simulink library "lib_energy_storage"  (Simulink 7.9)
settings: Solver=ode45  SolverMode=SingleTasking  StartTime=0.0  StopTime=10.0  RelTol=1e-3
undefined symbols (not defined in the file or in its folder): air_cp, amb_tmp, cyc_mph, enable_stop, ess_cap, ess_cap_scale, ess_cb, ess_cc, ess_coulombic_eff, ess_init_soc, ess_max_ah_cap, ess_max_p, ess_max_p_soc, ess_max_soc, ess_max_volts, ess_min_soc, ess_min_volts, ess_MMi, ess_MMo, ess_mod_airflow, ess_mod_cp, ess_mod_cpm, ess_mod_init_tmp, ess_module_mass, ess_module_num, ess_on, ess_parallel_mod_num, ess_r, ess_r_chg, ess_r_dis, ess_rc, ess_re, ess_res_scale_coef, ess_res_scale_fun, ess_rt, ess_set_tmp, ess_soc, ess_th_calc, ess_th_res, ess_th_res_off, ess_th_res_on, ess_tmp, ess_voc, fund_byu, fund_byuop, mc_min_volts, saber_air_temp, Saber_Battery_IO_File, saber_init_soc, saber_init_temp, saber_init_voc, saber_k_cb, saber_k_cc, saber_k_rc, saber_k_re, saber_k_rt, saber_k_soc, t_soc, time_step
libraries: lib_energy_storage x3
(part 2 of 3)

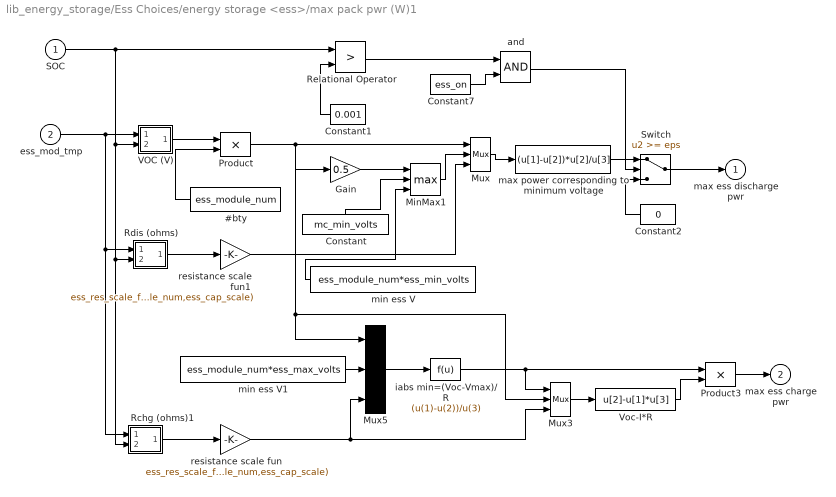
== system lib_energy_storage/Ess Choices/energy storage <ess>/max pack pwr (W)1 ==
  SOC : Inport
  ess_mod_tmp : Inport  Port=2
  #bty : Constant  Value=ess_module_num
  Constant : Constant  Value=mc_min_volts
  Constant1 : Constant  Value=0.001
  Constant2 : Constant  Value=0
  Constant7 : Constant  Value=ess_on
  Gain : Gain  Gain=0.5  SaturateOnIntegerOverflow=on  OutDataTypeStr=Inherit: Same as input  ParamDataTypeStr=Inherit: Same as input
  MinMax1 : MinMax  Function=max  Inputs=3  SaturateOnIntegerOverflow=on  InputSameDT=on
  Mux : Mux  Inputs=3
  Mux3 : Mux  Inputs=3
  Mux5 : Mux  Inputs=3
  Product : Product  SaturateOnIntegerOverflow=on  RndMeth=Zero  InputSameDT=on  OutDataTypeStr=Inherit: Same as first input
  Product3 : Product  SaturateOnIntegerOverflow=on  RndMeth=Zero  InputSameDT=on  OutDataTypeStr=Inherit: Same as first input
  Rchg (ohms)1 : Subsystem  mask(2-D Table Lookup){xindex=ess_tmp, yindex=ess_soc, table=ess_r_chg}
      mask prompts: xindex "X Index"; yindex "Y Index"
      mask help:
      | Two Dimensional Table Lookup
      | The first input corresponds to X Index and the second input corresponds to the Y Index
      mask init:
      | sftab2chk(xindex,yindex,table);
      mask Help: This block returns a linearly interpolated intersection from the table using the X index (which corresponds to the rows of the table) and the Y index (which corresponds to the columns of the table).  Extrapolation is used.
      mask Display: plot(-10,-10,110,110,[90,50,10],[90,40,30],[90,50,10],[50,26,20],[90,50,10],[22,13,10])
  Rdis (ohms) : Subsystem  mask(2-D Table Lookup){xindex=ess_tmp, yindex=ess_soc, table=ess_r_dis}
      mask prompts: xindex "X Index"; yindex "Y Index"
      mask help:
      | Two Dimensional Table Lookup
      | The first input corresponds to X Index and the second input corresponds to the Y Index
      mask init:
      | sftab2chk(xindex,yindex,table);
      mask Help: This block returns a linearly interpolated intersection from the table using the X index (which corresponds to the rows of the table) and the Y index (which corresponds to the columns of the table).  Extrapolation is used.
      mask Display: plot(-10,-10,110,110,[90,50,10],[90,40,30],[90,50,10],[50,26,20],[90,50,10],[22,13,10])
  Relational Operator : RelationalOperator  Operator=>  InputSameDT=on
  Switch : Switch  Threshold=eps  SaturateOnIntegerOverflow=on  InputSameDT=on
  VOC (V) : Subsystem  mask(2-D Table Lookup){xindex=ess_tmp, yindex=ess_soc, table=ess_voc}
      mask prompts: xindex "X Index"; yindex "Y Index"
      mask help:
      | Two Dimensional Table Lookup
      | The first input corresponds to X Index and the second input corresponds to the Y Index
      mask init:
      | sftab2chk(xindex,yindex,table);
      mask Help: This block returns a linearly interpolated intersection from the table using the X index (which corresponds to the rows of the table) and the Y index (which corresponds to the columns of the table).  Extrapolation is used.
      mask Display: plot(-10,-10,110,110,[90,50,10],[90,40,30],[90,50,10],[50,26,20],[90,50,10],[22,13,10])
  Voc-I*R : Fcn  Expr=u[2]-u[1]*u[3]
  and : Logic
  iabs min=(Voc-Vmax)/R : Fcn  Expr=(u(1)-u(2))/u(3)
  max power corresponding to minimum voltage : Fcn  Expr=(u[1]-u[2])*u[2]/u[3]
  min ess V : Constant  Value=ess_module_num*ess_min_volts
  min ess V1 : Constant  Value=ess_module_num*ess_max_volts
  resistance scale fun : Gain  Gain=ess_res_scale_fun(ess_res_scale_coef,ess_module_num,ess_cap_scale)  SaturateOnIntegerOverflow=on  OutDataTypeStr=Inherit: Same as input  ParamDataTypeStr=Inherit: Same as input
  resistance scale fun1 : Gain  Gain=ess_res_scale_fun(ess_res_scale_coef,ess_module_num,ess_cap_scale)  SaturateOnIntegerOverflow=on  OutDataTypeStr=Inherit: Same as input  ParamDataTypeStr=Inherit: Same as input
  max ess discharge pwr : Outport  InitialOutput=0
  max ess charge pwr : Outport  Port=2  InitialOutput=0
  wires:
  Constant7/1 -> and/2
  Relational Operator/1 -> and/1
  and/1 -> Switch/2
  min ess V/1 -> MinMax1/3
  ess_mod_tmp/1 -> VOC (V)/1(x0), Rdis (ohms)/1(x0), Rchg (ohms)1/1(x0)
  Constant1/1 -> Relational Operator/2
  Constant/1 -> MinMax1/2
  Mux/1 -> max power corresponding to minimum voltage/1
  Gain/1 -> MinMax1/1
  MinMax1/1 -> Mux/2
  Product/1 -> Mux/1, Gain/1, Mux5/1, Mux3/2
  resistance scale fun1/1 -> Mux/3
  VOC (V)/1(table out) -> Product/1
  Rdis (ohms)/1(table out) -> resistance scale fun1/1
  max power corresponding to minimum voltage/1 -> Switch/1
  Constant2/1 -> Switch/3
  SOC/1 -> Relational Operator/1, VOC (V)/2(y0), Rdis (ohms)/2(y0), Rchg (ohms)1/2(y0)
  Switch/1 -> max ess discharge pwr/1
  min ess V1/1 -> Mux5/2
  Mux5/1 -> iabs min=(Voc-Vmax)/R/1
  Mux3/1 -> Voc-I*R/1
  iabs min=(Voc-Vmax)/R/1 -> Mux3/1, Product3/1
  Voc-I*R/1 -> Product3/2
  Product3/1 -> max ess charge pwr/1
  resistance scale fun/1 -> Mux5/3, Mux3/3
  Rchg (ohms)1/1(table out) -> resistance scale fun/1
  #bty/1 -> Product/2

== system lib_energy_storage/Ess Choices/energy storage <ess>/pack Voc, Rint ==
  SOC (prev) : Inport
  req'd battery power (W) : Inport  Port=2
  mod tmp   (C) : Inport  Port=3
  #bty : Constant  Value=ess_module_num
  Product : Product  SaturateOnIntegerOverflow=on  RndMeth=Zero  InputSameDT=on  OutDataTypeStr=Inherit: Same as first input
  Rchg (ohms) : Subsystem  mask(2-D Table Lookup){xindex=ess_tmp, yindex=ess_soc, table=ess_r_chg}
      mask prompts: xindex "X Index"; yindex "Y Index"
      mask help:
      | Two Dimensional Table Lookup
      | The first input corresponds to X Index and the second input corresponds to the Y Index
      mask init:
      | sftab2chk(xindex,yindex,table);
      mask Help: This block returns a linearly interpolated intersection from the table using the X index (which corresponds to the rows of the table) and the Y index (which corresponds to the columns of the table).  Extrapolation is used.
      mask Display: plot(-10,-10,110,110,[90,50,10],[90,40,30],[90,50,10],[50,26,20],[90,50,10],[22,13,10])
  Rdis (ohms) : Subsystem  mask(2-D Table Lookup){xindex=ess_tmp, yindex=ess_soc, table=ess_r_dis}
      mask prompts: xindex "X Index"; yindex "Y Index"
      mask help:
      | Two Dimensional Table Lookup
      | The first input corresponds to X Index and the second input corresponds to the Y Index
      mask init:
      | sftab2chk(xindex,yindex,table);
      mask Help: This block returns a linearly interpolated intersection from the table using the X index (which corresponds to the rows of the table) and the Y index (which corresponds to the columns of the table).  Extrapolation is used.
      mask Display: plot(-10,-10,110,110,[90,50,10],[90,40,30],[90,50,10],[50,26,20],[90,50,10],[22,13,10])
  Switch : Switch  SaturateOnIntegerOverflow=on  InputSameDT=on
  VOC (V) : Subsystem  mask(2-D Table Lookup){xindex=ess_tmp, yindex=ess_soc, table=ess_voc}
      mask prompts: xindex "X Index"; yindex "Y Index"
      mask help:
      | Two Dimensional Table Lookup
      | The first input corresponds to X Index and the second input corresponds to the Y Index
      mask init:
      | sftab2chk(xindex,yindex,table);
      mask Help: This block returns a linearly interpolated intersection from the table using the X index (which corresponds to the rows of the table) and the Y index (which corresponds to the columns of the table).  Extrapolation is used.
      mask Display: plot(-10,-10,110,110,[90,50,10],[90,40,30],[90,50,10],[50,26,20],[90,50,10],[22,13,10])
  resistance scale fun : Gain  Gain=ess_res_scale_fun(ess_res_scale_coef,ess_module_num,ess_cap_scale)  SaturateOnIntegerOverflow=on  OutDataTypeStr=Inherit: Same as input  ParamDataTypeStr=Inherit: Same as input
  resistance scale fun1 : Gain  Gain=ess_res_scale_fun(ess_res_scale_coef,ess_module_num,ess_cap_scale)  SaturateOnIntegerOverflow=on  OutDataTypeStr=Inherit: Same as input  ParamDataTypeStr=Inherit: Same as input
  pack open- circuit voltage : Outport  InitialOutput=0
  pack resistance : Outport  Port=2  InitialOutput=0
  wires:
  mod tmp   (C)/1 -> Rchg (ohms)/1(x0), Rdis (ohms)/1(x0), VOC (V)/1(x0)
  SOC (prev)/1 -> Rchg (ohms)/2(y0), Rdis (ohms)/2(y0), VOC (V)/2(y0)
  req'd battery power (W)/1 -> Switch/2
  VOC (V)/1(table out) -> Product/1
  Product/1 -> pack open- circuit voltage/1
  #bty/1 -> Product/2
  Switch/1 -> pack resistance/1
  Rdis (ohms)/1(table out) -> resistance scale fun/1
  resistance scale fun/1 -> Switch/1
  Rchg (ohms)/1(table out) -> resistance scale fun1/1
  resistance scale fun1/1 -> Switch/3

== system lib_energy_storage/Ess Choices/energy storage <ess>/stop sim ==
  SOC : Inport
  Enable : EnablePort
  Const : Constant  Value=.001
  Relational Operator : RelationalOperator  Operator=<  InputSameDT=on
  Stop Simulation : Stop
  wires:
  Relational Operator/1 -> Stop Simulation/1
  SOC/1 -> Relational Operator/1
  Const/1 -> Relational Operator/2

== system lib_energy_storage/Ess Choices/energy storage <ess> RC/Allow simulation to stop based on  low SOC ==
  SOC : Inport
  Enable : EnablePort
  Const : Constant  Value=.001
  Relational Operator : RelationalOperator  Operator=<  InputSameDT=on
  Stop Simulation : Stop
  wires:
  Relational Operator/1 -> Stop Simulation/1
  SOC/1 -> Relational Operator/1
  Const/1 -> Relational Operator/2

== system lib_energy_storage/Ess Choices/energy storage <ess> RC/Block NOTES ==
  note: This block models the energy storage system as an SOC-dependent voltage
      | in series with an SOC- and current direction-dependent internal resistance.
      | SOC is computed assuming that A-h capacity is constant, but limited
      | such that a minimum voltage is never exceeded (replacing the
      | previous Peukert relationship which underpredicted battery capacity).
      |
      | Discharge power is limited here so as not to bring the bus (battery pack) voltage below
      | the minimum controller voltage or the minimum battery voltage and so as to allow
      | the solution of the quadratic eq'n for discharge current.
      |
      | Charge current is limited to ensure the voltage does not exceed a maximum
      | voltage
      |
      | Positive current is discharge current in the convention used here.
      | Power loss is computed as I*R+losses due to Coulombic (in)efficiency.
      |
      | Thermal modeling of the battery performance is modeled in the
      | OCV, Rint, and capacity.

== system lib_energy_storage/Ess Choices/energy storage <ess> RC/Model Parameters ==
  SOC : Inport
  Ess Temp : Inport  Port=2
  Preq : Inport  Port=3
  Terminator : Terminator
  cb : Lookup  InputValues=ess_tmp  Table=ess_cb  SaturateOnIntegerOverflow=on
  cc : Lookup  InputValues=ess_tmp  Table=ess_cc  SaturateOnIntegerOverflow=on
  rc : Subsystem  mask(2-D Table Lookup){xindex=ess_tmp, yindex=ess_soc, table=ess_rc}
      mask prompts: xindex "X Index"; yindex "Y Index"
      mask help:
      | Two Dimensional Table Lookup
      | The first input corresponds to X Index and the second input corresponds to the Y Index
      mask init:
      | sftab2chk(xindex,yindex,table);
      mask Help: This block returns a linearly interpolated intersection from the table using the X index (which corresponds to the rows of the table) and the Y index (which corresponds to the columns of the table).  Extrapolation is used.
      mask Display: plot(-10,-10,110,110,[90,50,10],[90,40,30],[90,50,10],[50,26,20],[90,50,10],[22,13,10])
  re : Subsystem  mask(2-D Table Lookup){xindex=ess_tmp, yindex=ess_soc, table=ess_re}
      mask prompts: xindex "X Index"; yindex "Y Index"
      mask help:
      | Two Dimensional Table Lookup
      | The first input corresponds to X Index and the second input corresponds to the Y Index
      mask init:
      | sftab2chk(xindex,yindex,table);
      mask Help: This block returns a linearly interpolated intersection from the table using the X index (which corresponds to the rows of the table) and the Y index (which corresponds to the columns of the table).  Extrapolation is used.
      mask Display: plot(-10,-10,110,110,[90,50,10],[90,40,30],[90,50,10],[50,26,20],[90,50,10],[22,13,10])
  rt : Subsystem  mask(2-D Table Lookup){xindex=ess_tmp, yindex=ess_soc, table=ess_rt}
      mask prompts: xindex "X Index"; yindex "Y Index"
      mask help:
      | Two Dimensional Table Lookup
      | The first input corresponds to X Index and the second input corresponds to the Y Index
      mask init:
      | sftab2chk(xindex,yindex,table);
      mask Help: This block returns a linearly interpolated intersection from the table using the X index (which corresponds to the rows of the table) and the Y index (which corresponds to the columns of the table).  Extrapolation is used.
      mask Display: plot(-10,-10,110,110,[90,50,10],[90,40,30],[90,50,10],[50,26,20],[90,50,10],[22,13,10])
  Cb : Outport  InitialOutput=0
  Cc : Outport  Port=2  InitialOutput=0
  Re : Outport  Port=3  InitialOutput=0
  Rc : Outport  Port=4  InitialOutput=0
  Rt : Outport  Port=5  InitialOutput=0
  wires:
  rc/1(table out) -> Rc/1
  rt/1(table out) -> Rt/1
  re/1(table out) -> Re/1
  cc/1 -> Cc/1
  cb/1 -> Cb/1
  SOC/1 -> rt/2(y0), rc/2(y0), re/2(y0)
  Preq/1 -> Terminator/1
  Ess Temp/1 -> rt/1(x0), rc/1(x0), re/1(x0), cc/1, cb/1

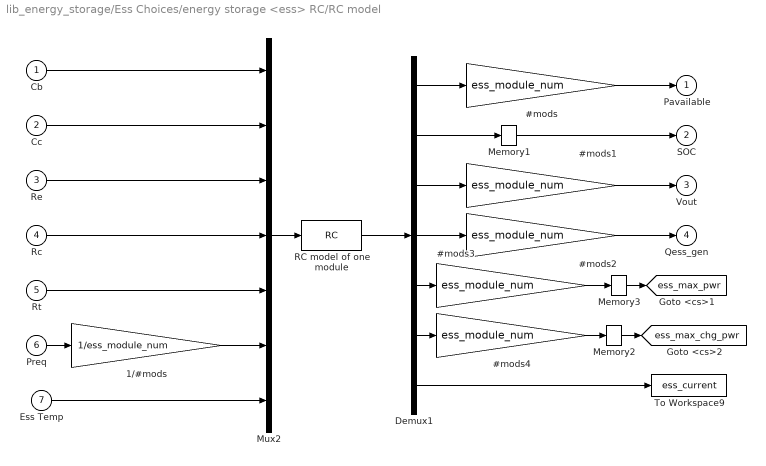
== system lib_energy_storage/Ess Choices/energy storage <ess> RC/RC model ==
  Cb : Inport
  Cc : Inport  Port=2
  Re : Inport  Port=3
  Rc : Inport  Port=4
  Rt : Inport  Port=5
  Preq : Inport  Port=6
  Ess Temp : Inport  Port=7
  #mods{,1..4} (5 alike) : Gain  Gain=ess_module_num  SaturateOnIntegerOverflow=on  OutDataTypeStr=Inherit: Same as input  ParamDataTypeStr=Inherit: Same as input
  1/#mods : Gain  Gain=1/ess_module_num  SaturateOnIntegerOverflow=on  OutDataTypeStr=Inherit: Same as input  ParamDataTypeStr=Inherit: Same as input
  Demux1 : Demux  Outputs=7
  Memory1 : Memory  X0=ess_init_soc
  Memory2 : Memory
  Memory3 : Memory
  Mux2 : Mux  Inputs=7
  RC model of one module : S-Function  FunctionName=RC  Parameters=ess_min_volts,ess_max_volts,mc_min_volts/ess_module_num,ess_soc,ess_tmp,ess_voc,ess_init_soc,ess_mod_init_tmp  EnableBusSupport=off
  To Workspace9 : ToWorkspace  VariableName=ess_current  SampleTime=-1
  Pavailable : Outport  InitialOutput=0
  SOC : Outport  Port=2  InitialOutput=0
  Vout : Outport  Port=3  InitialOutput=0
  Qess_gen : Outport  Port=4  InitialOutput=0
  tag scope: ess_max_chg_pwr=global, ess_max_pwr=global
  wires:
  RC model of one module/1 -> Demux1/1
  #mods2/1 -> Qess_gen/1
  Demux1/4 -> #mods2/1
  #mods1/1 -> Vout/1
  Demux1/3 -> #mods1/1
  #mods/1 -> Pavailable/1
  Demux1/1 -> #mods/1
  1/#mods/1 -> Mux2/6
  Preq/1 -> 1/#mods/1
  Mux2/1 -> RC model of one module/1
  Rt/1 -> Mux2/5
  Rc/1 -> Mux2/4
  Re/1 -> Mux2/3
  Cc/1 -> Mux2/2
  Cb/1 -> Mux2/1
  Ess Temp/1 -> Mux2/7
  Demux1/7 -> To Workspace9/1
  Demux1/6 -> #mods4/1
  Memory2/1 -> [ess_max_chg_pwr]
  Demux1/5 -> #mods3/1
  Memory3/1 -> [ess_max_pwr]
  Demux1/2 -> Memory1/1
  Memory1/1 -> SOC/1
  #mods3/1 -> Memory3/1
  #mods4/1 -> Memory2/1

== system lib_energy_storage/Ess Choices/energy storage <ess> RC/Thermal Model of Battery ==
  Qess_gen : Inport
  Enable : EnablePort  StatesWhenEnabling=reset
  #of mods : Gain  Gain=ess_module_num  SaturateOnIntegerOverflow=on  OutDataTypeStr=Inherit: Same as input  ParamDataTypeStr=Inherit: Same as input
  1/#of mods : Gain  Gain=1/ess_module_num  SaturateOnIntegerOverflow=on  OutDataTypeStr=Inherit: Same as input  ParamDataTypeStr=Inherit: Same as input
  1/mcp : Gain  Gain=1/(ess_module_mass*ess_mod_cp)  SaturateOnIntegerOverflow=on  OutDataTypeStr=Inherit: Same as input  ParamDataTypeStr=Inherit: Same as input
  Block NOTES : Subsystem
      mask Display: disp('Block\nNOTES')
  Memory : Memory  X0=cyc_mph(1,2)*.447
  Memory1 : Memory  X0=cyc_mph(1,2)*.447
  Mux20 : Mux  Inputs=3
  Qc : Sum  SaturateOnIntegerOverflow=on  InputSameDT=on  OutDataTypeStr=Inherit: Same as first input
  Qess_case : Fcn  Expr=(u(2) - u(1))/u(3)
  Saturation3 : Saturate  UpperLimit=1  LowerLimit=0
  Tair,ave : Subsystem  TreatAsAtomicUnit=on
  Tess2 : Integrator  InitialCondition=ess_mod_init_tmp
  thermostat : Fcn  Expr=u(1) - ess_set_tmp
  Tess : Outport  InitialOutput=0
  Tair : Outport  Port=2
  Qair : Outport  Port=3  OutputWhenDisabled=reset  InitialOutput=0
  wires:
  Tair,ave/1(Tair_ave) -> Tair/1, Mux20/2
  Tair,ave/2(Th Res) -> Mux20/3
  Mux20/1 -> Qess_case/1
  #of mods/1 -> Qair/1
  Memory/1 -> Tair,ave/1(Qess_case)
  Memory1/1 -> Tair,ave/Enable
  Saturation3/1 -> Memory1/1
  thermostat/1 -> Saturation3/1
  1/#of mods/1 -> Qc/2
  Qess_gen/1 -> 1/#of mods/1
  Tess2/1 -> thermostat/1, Mux20/1, Tess/1
  1/mcp/1 -> Tess2/1
  Qess_case/1 -> #of mods/1, Memory/1, Qc/1
  Qc/1 -> 1/mcp/1

== system lib_energy_storage/Ess Choices/energy storage <ess> RC/documentation9 ==

== system lib_energy_storage/Ess Choices/energy storage <ess> nnet/Limits ==
  power req : Inport
  power  available from battery : Inport  Port=2
  Const{1..4} (4 alike) : Constant  Value=0
  Relational Operator1 : RelationalOperator  Operator===  InputSameDT=on
  limited by battery : Logic  Operator=NOT  Inputs=1
  tag scope: ess_maxV_limited=global, ess_minV_limited=global, ess_pwr_limited=global, ess_soc_limited=global, mc_voltage_limited=global
  wires:
  Relational Operator1/1 -> limited by battery/1
  limited by battery/1 -> [ess_pwr_limited]
  power req/1 -> Relational Operator1/1
  power  available from battery/1 -> Relational Operator1/2
  Const4/1 -> [mc_voltage_limited]
  Const3/1 -> [ess_minV_limited]
  Const2/1 -> [ess_maxV_limited]
  Const1/1 -> [ess_soc_limited]

== system lib_energy_storage/Ess Choices/energy storage <ess> nnet/NNet ==
  Preq : Inport
  SOC : Inport  Port=2
  Enable : EnablePort
  De-Normalizer1 Voltage : Fcn  Expr=(u-0.2)*(ess_MMo(2,2)-ess_MMo(2,1))/(0.8-0.2)+ess_MMo(2,1)
  De-Normalizer2 Current : Fcn  Expr=(u-0.2)*(ess_MMo(1,2)-ess_MMo(1,1))/(0.8-0.2)+ess_MMo(1,1)
  Demux : Demux  Outputs=2
  Mux : Mux  Inputs=2
  Neural Network : Subsystem
  Normalizer Power : Fcn  Expr=(u-ess_MMi(1,1))/(ess_MMi(1,2)-ess_MMi(1,1))
  Normalizer SOC : Fcn  Expr=(u-ess_MMi(2,1))/(ess_MMi(2,2)-ess_MMi(2,1))
  V : Outport  InitialOutput=0
  i : Outport  Port=2  OutputWhenDisabled=reset  InitialOutput=0
  wires:
  De-Normalizer1 Voltage/1 -> V/1
  Demux/2 -> De-Normalizer1 Voltage/1
  Demux/1 -> De-Normalizer2 Current/1
  De-Normalizer2 Current/1 -> i/1
  Normalizer SOC/1 -> Mux/2
  SOC/1 -> Normalizer SOC/1
  Normalizer Power/1 -> Mux/1
  Preq/1 -> Normalizer Power/1
  Neural Network/1("y{1}") -> Demux/1
  Mux/1 -> Neural Network/1("p{1}")

== system lib_energy_storage/Ess Choices/energy storage <ess> nnet/No Thermal model ==
  Const1 : Constant  Value=0
  Const2 : Constant  Value=amb_tmp
  Const3 : Constant  Value=0
  To WS1 : ToWorkspace  VariableName=ess_pwr_loss_a
  To WS2 : ToWorkspace  VariableName=ess_mod_tmp
  To WS3 : ToWorkspace  VariableName=ess_air_tmp
  To WS4 : ToWorkspace  VariableName=ess_air_th_pwr
  wires:
  Const3/1 -> To WS4/1
  Const2/1 -> To WS3/1, To WS2/1
  Const1/1 -> To WS1/1

== system lib_energy_storage/Ess Choices/energy storage <ess> nnet/SOC algorithm ==
  note: SOC=(Max Ah capacity-Ah used)/Max Ah capacity
  (A) : Inport
  tmp (C) : Inport  Port=2
  (sec->hrs) : Gain  Gain=1/3600  SaturateOnIntegerOverflow=on  OutDataTypeStr=Inherit: Same as input  ParamDataTypeStr=Inherit: Same as input
  0 <= SOC <= 1 : Saturate  UpperLimit=1  LowerLimit=0
  A-h remaining : Sum  Inputs=-+  SaturateOnIntegerOverflow=on  InputSameDT=on  OutDataTypeStr=Inherit: Same as first input
  Ah used : Integrator  InitialConditionSource=external  InitialCondition=(1-ess_init_soc)*ess_max_ah_cap
  Fcn : Fcn  Expr=1/u
  Fcn1 : Fcn  Expr=(1-ess_init_soc)*u
  SOC : Product  SaturateOnIntegerOverflow=on  RndMeth=Zero  InputSameDT=on  OutDataTypeStr=Inherit: Same as first input
  Switch : Switch  SaturateOnIntegerOverflow=on  InputSameDT=on
  adjusted A : Product  SaturateOnIntegerOverflow=on  RndMeth=Zero  InputSameDT=on  OutDataTypeStr=Inherit: Same as first input
  coul eff : Lookup  InputValues=ess_tmp  Table=ess_coulombic_eff  SaturateOnIntegerOverflow=on
  max cap : Lookup  InputValues=ess_tmp  Table=ess_max_ah_cap  SaturateOnIntegerOverflow=on
  SOC1 : Outport  InitialOutput=0
  wires:
  Fcn1/1 -> Ah used/2
  max cap/1 -> Fcn1/1, Fcn/1, A-h remaining/2
  adjusted A/1 -> Switch/3
  coul eff/1 -> adjusted A/2
  tmp (C)/1 -> coul eff/1, max cap/1
  0 <= SOC <= 1/1 -> SOC1/1
  A-h remaining/1 -> SOC/1
  SOC/1 -> 0 <= SOC <= 1/1
  Fcn/1 -> SOC/2
  Ah used/1 -> A-h remaining/1
  (sec->hrs)/1 -> Ah used/1
  Switch/1 -> (sec->hrs)/1
  (A)/1 -> adjusted A/1, Switch/1, Switch/2

== system lib_energy_storage/Ess Choices/energy storage <ess> nnet/max pack pwr (W) ==
  SOC : Inport
  # batteries : Gain  Gain=ess_module_num  SaturateOnIntegerOverflow=on  OutDataTypeStr=Inherit: Same as input  ParamDataTypeStr=Inherit: Same as input
  max power : Lookup  InputValues=ess_max_p_soc  Table=ess_max_p  SaturateOnIntegerOverflow=on
  ess discharge pwr : Outport  InitialOutput=0
  wires:
  # batteries/1 -> ess discharge pwr/1
  max power/1 -> # batteries/1
  SOC/1 -> max power/1

== system lib_energy_storage/Ess Choices/energy storage <ess> nnet/stop sim ==
  SOC : Inport
  Enable : EnablePort
  Const : Constant  Value=.001
  Relational Operator : RelationalOperator  Operator=<  InputSameDT=on
  Stop Simulation : Stop
  wires:
  Relational Operator/1 -> Stop Simulation/1
  SOC/1 -> Relational Operator/1
  Const/1 -> Relational Operator/2

== system lib_energy_storage/Ess Choices/energy storage <ess> Saber/Block NOTES ==
  note: Saber co-simulation

== system lib_energy_storage/Ess Choices/energy storage <ess> Saber/Power ==
  Current : Inport
  Voltage : Inport  Port=2
  P=i*V : Product  SaturateOnIntegerOverflow=on  RndMeth=Zero  InputSameDT=on  OutDataTypeStr=Inherit: Same as first input
  To Workspace9 : ToWorkspace  VariableName=ess_pwr_out_a  SampleTime=-1
  Avail Power : Outport
  wires:
  P=i*V/1 -> Avail Power/1, To Workspace9/1
  Current/1 -> P=i*V/1
  Voltage/1 -> P=i*V/2

== system lib_energy_storage/Ess Choices/energy storage <ess> Saber/Power request ==
  power req'd : Inport
  1/# batteries : Gain  Gain=1/ess_module_num  SaturateOnIntegerOverflow=on  OutDataTypeStr=Inherit: Same as input  ParamDataTypeStr=Inherit: Same as input
  Relational Operator1 : RelationalOperator  Operator===  InputSameDT=on
  To Workspace8 : ToWorkspace  VariableName=ess_pwr_out_r  SampleTime=-1
  if P==0 : Constant  Value=0
  "if P==0, pass  P=0.0001" : Switch  Threshold=0.1  SaturateOnIntegerOverflow=on  InputSameDT=on
  non-zero power : Constant  Value=0.0001
  P request : Outport
  wires:
  power req'd/1 -> To Workspace8/1, 1/# batteries/1
  1/# batteries/1 -> "if P==0, pass  P=0.0001"/3, Relational Operator1/2
  "if P==0, pass  P=0.0001"/1 -> P request/1
  if P==0/1 -> Relational Operator1/1
  non-zero power/1 -> "if P==0, pass  P=0.0001"/1
  Relational Operator1/1 -> "if P==0, pass  P=0.0001"/2

== system lib_energy_storage/Ess Choices/energy storage <ess> Saber/SOC's ==
  Saber SOC's : Inport
  Const : Constant  Value=enable_stop
  Mean : Subsystem
  To Workspace2 : ToWorkspace  VariableName=saber_ess_SOC  SampleTime=-1
  soc mem : Memory  X0=ess_init_soc
  stop sim : Subsystem  TreatAsAtomicUnit=on
  tag scope: SOC=global
  wires:
  Saber SOC's/1 -> Mean/1(In), To Workspace2/1
  Const/1 -> stop sim/Enable
  Mean/1(Out) -> soc mem/1
  soc mem/1 -> [SOC], stop sim/1(SOC)

== system lib_energy_storage/Ess Choices/energy storage <ess> Saber/Temps ==
  Saber Temps : Inport
  Mean : Subsystem
  To WS2 : ToWorkspace  VariableName=ess_mod_tmp
  To Workspace3 : ToWorkspace  VariableName=saber_ess_temp  SampleTime=-1
  wires:
  Saber Temps/1 -> Mean/1(In), To Workspace3/1
  Mean/1(Out) -> To WS2/1

== system lib_energy_storage/Ess Choices/energy storage <ess> Saber/Thermal Power ==
  Saber Thermal P : Inport
  # batteries : Gain  Gain=ess_module_num  SaturateOnIntegerOverflow=on  OutDataTypeStr=Inherit: Same as input  ParamDataTypeStr=Inherit: Same as input
  Saturation : Saturate  UpperLimit=inf  LowerLimit=0
  Sum2 : Sum  Inputs=1  SaturateOnIntegerOverflow=on  InputSameDT=on  OutDataTypeStr=Inherit: Same as first input
  To Workspace3 : ToWorkspace  VariableName=saber_ess_th_pwr  SampleTime=-1
  To Workspace9 : ToWorkspace  VariableName=ess_pwr_loss_a  SampleTime=-1
  wires:
  Sum2/1 -> To Workspace9/1
  # batteries/1 -> Sum2/1, To Workspace3/1
  Saber Thermal P/1 -> Saturation/1
  Saturation/1 -> # batteries/1

== system lib_energy_storage/Ess Choices/energy storage <ess> Saber/Time Dependent Power Request ==
  P request : Inport
  Constant : Constant  Value=0
  Enabled Subsystem1 : Subsystem  TreatAsAtomicUnit=on
  IC : InitialCondition  Value=time_step
  Matrix Concatenation1 : lib_energy_storage/Ess Choices/energy storage <ess> Saber/Matrix Concatenation1  numInports=6  catMethod=Horizontal
  Memory1 : Memory  X0=.001  InheritSampleTime=on
  Memory2 : Memory  X0=80  InheritSampleTime=on
  Relational Operator : RelationalOperator  Operator===  InputSameDT=on
  Saturation : Saturate  UpperLimit=inf  LowerLimit=.001
  P request time : Outport
  wires:
  Relational Operator/1 -> Enabled Subsystem1/Enable
  [time] -> Relational Operator/2
  Enabled Subsystem1/1(Out1) -> Matrix Concatenation1/2
  Memory2/1 -> Matrix Concatenation1/4
  Matrix Concatenation1/1 -> P request time/1
  IC/1 -> Matrix Concatenation1/5
  Saturation/1 -> Memory1/1
  [time] -> Saturation/1
  Memory1/1 -> Matrix Concatenation1/3
  [time] -> IC/1
  Constant/1 -> Relational Operator/1, Matrix Concatenation1/1
  P request/1 -> Memory2/1, Matrix Concatenation1/6, Enabled Subsystem1/1(In1)  "P request"

== system lib_energy_storage/Ess Choices/energy storage <ess> Saber/Voltages ==
  Saber Voltages : Inport
  # batteries : Gain  Gain=ess_module_num  SaturateOnIntegerOverflow=on  OutDataTypeStr=Inherit: Same as input  ParamDataTypeStr=Inherit: Same as input
  Sum : Sum  Inputs=1  SaturateOnIntegerOverflow=on  InputSameDT=on  OutDataTypeStr=Inherit: Same as first input
  To Workspace1 : ToWorkspace  VariableName=ess_voltage  SampleTime=-1
  To Workspace11 : ToWorkspace  VariableName=saber_ess_voltage  SampleTime=-1
  ADV Voltage : Outport
  tag scope: bus_voltage=global
  wires:
  # batteries/1 -> Sum/1, To Workspace11/1
  Sum/1 -> [bus_voltage], To Workspace1/1, ADV Voltage/1
  Saber Voltages/1 -> # batteries/1

== system lib_energy_storage/Ess Choices/energy storage <ess> Saber/max pack pwr (W) ==
  note: Edit in the future
      | Used in series power follower
  Ground : Ground
  tag scope: ess_max_pwr=global
  wires:
  Ground/1 -> [ess_max_pwr]

== system lib_energy_storage/Ess Choices/energy storage <ess> fundamental model/Block NOTES ==
  note: Fundamentally based SOC model developed at BYU
      | Files needed:
      | input1.dat
      | input2.dat
      | input3.dat
      | nrel13cs.dll

== system lib_energy_storage/Ess Choices/energy storage <ess> fundamental model/ess tmp ==
  Qess_gen : Inport
  Enable : EnablePort  StatesWhenEnabling=reset
  #of mods : Gain  Gain=ess_module_num  SaturateOnIntegerOverflow=on  OutDataTypeStr=Inherit: Same as input  ParamDataTypeStr=Inherit: Same as input
  1/#of mods : Gain  Gain=1/ess_module_num  SaturateOnIntegerOverflow=on  OutDataTypeStr=Inherit: Same as input  ParamDataTypeStr=Inherit: Same as input
  1/mcp : Gain  Gain=1/(ess_module_mass*ess_mod_cp)  SaturateOnIntegerOverflow=on  OutDataTypeStr=Inherit: Same as input  ParamDataTypeStr=Inherit: Same as input
  Block NOTES : Subsystem
      mask Display: disp('Block\nNOTES')
  Memory : Memory  X0=cyc_mph(1,2)*.447
  Memory1 : Memory  X0=cyc_mph(1,2)*.447
  Mux20 : Mux  Inputs=3
  Qc : Sum  SaturateOnIntegerOverflow=on  InputSameDT=on  OutDataTypeStr=Inherit: Same as first input
  Qess_case : Fcn  Expr=(u(2) - u(1))/u(3)
  Saturation3 : Saturate  UpperLimit=1  LowerLimit=0
  Tair,ave : Subsystem  TreatAsAtomicUnit=on
  Tess2 : Integrator  InitialCondition=ess_mod_init_tmp
  thermostat : Fcn  Expr=u(1) - ess_set_tmp
  Tess : Outport  InitialOutput=0
  Tair : Outport  Port=2
  Qair : Outport  Port=3  OutputWhenDisabled=reset  InitialOutput=0
  wires:
  Tair,ave/1(Tair_ave) -> Tair/1, Mux20/2
  Tair,ave/2(Th Res) -> Mux20/3
  Mux20/1 -> Qess_case/1
  #of mods/1 -> Qair/1
  Memory/1 -> Tair,ave/1(Qess_case)
  Memory1/1 -> Tair,ave/Enable
  Saturation3/1 -> Memory1/1
  thermostat/1 -> Saturation3/1
  1/#of mods/1 -> Qc/2
  Qess_gen/1 -> 1/#of mods/1
  Tess2/1 -> thermostat/1, Mux20/1, Tess/1
  1/mcp/1 -> Tess2/1
  Qess_case/1 -> #of mods/1, Memory/1, Qc/1
  Qc/1 -> 1/mcp/1

== system lib_energy_storage/Ess Choices/energy storage <ess> fundamental model/max pack pwr (W) ==
  SOC : Inport
  # batteries : Gain  Gain=ess_module_num  SaturateOnIntegerOverflow=on  OutDataTypeStr=Inherit: Same as input  ParamDataTypeStr=Inherit: Same as input
  max power : Lookup  InputValues=ess_max_p_soc  Table=ess_max_p  SaturateOnIntegerOverflow=on
  ess discharge pwr : Outport  InitialOutput=0
  wires:
  # batteries/1 -> ess discharge pwr/1
  max power/1 -> # batteries/1
  SOC/1 -> max power/1

== system lib_energy_storage/Ess Choices/energy storage <ess> fundamental model/stop sim ==
  SOC : Inport
  Enable : EnablePort
  Const : Constant  Value=0.1
  Relational Operator : RelationalOperator  Operator=<  InputSameDT=on
  Stop Simulation : Stop
  wires:
  Relational Operator/1 -> Stop Simulation/1
  SOC/1 -> Relational Operator/1
  Const/1 -> Relational Operator/2

== system lib_energy_storage/Ess Choices/energy storage <ess> optima fundamental model/Block NOTES ==
  note: Fundamentally based SOC model developed at BYU
      | Files needed:
      | input1.dat
      | input2.dat
      | input3.dat
      | nrel13cs.dll

== system lib_energy_storage/Ess Choices/energy storage <ess> optima fundamental model/ess tmp ==
  Qess_gen : Inport
  Enable : EnablePort  StatesWhenEnabling=reset
  #of mods : Gain  Gain=ess_module_num  SaturateOnIntegerOverflow=on  OutDataTypeStr=Inherit: Same as input  ParamDataTypeStr=Inherit: Same as input
  1/#of mods : Gain  Gain=1/ess_module_num  SaturateOnIntegerOverflow=on  OutDataTypeStr=Inherit: Same as input  ParamDataTypeStr=Inherit: Same as input
  1/mcp : Gain  Gain=1/(ess_module_mass*ess_mod_cp)  SaturateOnIntegerOverflow=on  OutDataTypeStr=Inherit: Same as input  ParamDataTypeStr=Inherit: Same as input
  Block NOTES : Subsystem
      mask Display: disp('Block\nNOTES')
  Memory : Memory  X0=cyc_mph(1,2)*.447
  Memory1 : Memory  X0=cyc_mph(1,2)*.447
  Mux20 : Mux  Inputs=3
  Qc : Sum  SaturateOnIntegerOverflow=on  InputSameDT=on  OutDataTypeStr=Inherit: Same as first input
  Qess_case : Fcn  Expr=(u(2) - u(1))/u(3)
  Saturation3 : Saturate  UpperLimit=1  LowerLimit=0
  Tair,ave : Subsystem  TreatAsAtomicUnit=on
  Tess2 : Integrator  InitialCondition=ess_mod_init_tmp
  thermostat : Fcn  Expr=u(1) - ess_set_tmp
  Tess : Outport  InitialOutput=0
  Tair : Outport  Port=2
  Qair : Outport  Port=3  OutputWhenDisabled=reset  InitialOutput=0
  wires:
  Tair,ave/1(Tair_ave) -> Tair/1, Mux20/2
  Tair,ave/2(Th Res) -> Mux20/3
  Mux20/1 -> Qess_case/1
  #of mods/1 -> Qair/1
  Memory/1 -> Tair,ave/1(Qess_case)
  Memory1/1 -> Tair,ave/Enable
  Saturation3/1 -> Memory1/1
  thermostat/1 -> Saturation3/1
  1/#of mods/1 -> Qc/2
  Qess_gen/1 -> 1/#of mods/1
  Tess2/1 -> thermostat/1, Mux20/1, Tess/1
  1/mcp/1 -> Tess2/1
  Qess_case/1 -> #of mods/1, Memory/1, Qc/1
  Qc/1 -> 1/mcp/1

== system lib_energy_storage/Ess Choices/energy storage <ess> optima fundamental model/max pack pwr (W) ==
  SOC : Inport
  # batteries : Gain  Gain=ess_module_num  SaturateOnIntegerOverflow=on  OutDataTypeStr=Inherit: Same as input  ParamDataTypeStr=Inherit: Same as input
  max power : Lookup  InputValues=ess_max_p_soc  Table=ess_max_p  SaturateOnIntegerOverflow=on
  ess discharge pwr : Outport  InitialOutput=0
  wires:
  # batteries/1 -> ess discharge pwr/1
  max power/1 -> # batteries/1
  SOC/1 -> max power/1

== system lib_energy_storage/Ess Choices/energy storage <ess> optima fundamental model/stop sim ==
  SOC : Inport
  Enable : EnablePort
  Const : Constant  Value=.001
  Relational Operator : RelationalOperator  Operator=<  InputSameDT=on
  Stop Simulation : Stop
  wires:
  Relational Operator/1 -> Stop Simulation/1
  SOC/1 -> Relational Operator/1
  Const/1 -> Relational Operator/2

== system lib_energy_storage/Ess Choices/Ultracapacitor  System/Calc Iout/SOC limit ==
  SOC : Inport
  Pbty : Inport  Port=2
  Constant1 : Constant  Value=0.001
  Constant5 : Constant  Value=.999
  Constant9 : Constant  Value=0
  Logical Operator : Logic  Operator=OR
  Logical Operator1 : Logic
  Logical Operator2 : Logic  Operator=NOT  Inputs=1
  Relational Operator : RelationalOperator  Operator=>  InputSameDT=on
  Relational Operator3 : RelationalOperator  Operator=<  InputSameDT=on
  SOC>=.999 : RelationalOperator  InputSameDT=on
  charging (Preq is neg) : RelationalOperator  Operator=<  InputSameDT=on
  no power req if SOC<0 and trying  to discharge : Switch  Threshold=eps  SaturateOnIntegerOverflow=on  InputSameDT=on
  no power req if SOC>.999 and trying  to charge : Switch  Threshold=eps  SaturateOnIntegerOverflow=on  InputSameDT=on
  "Pbty, limited" : Outport  InitialOutput=0
  tag scope: ess_soc_hi_limited=global, ess_soc_low_limited=global
  wires:
  Constant1/1 -> Relational Operator/2
  Pbty/1 -> Relational Operator3/1, charging (Preq is neg)/1, no power req if SOC<0 and trying  to discharge/1
  Logical Operator/1 -> Logical Operator2/1, no power req if SOC<0 and trying  to discharge/2
  SOC/1 -> Relational Operator/1, SOC>=.999/1
  SOC>=.999/1 -> Logical Operator1/1
  charging (Preq is neg)/1 -> Logical Operator1/2
  Constant5/1 -> SOC>=.999/2
  no power req if SOC<0 and trying  to discharge/1 -> no power req if SOC>.999 and trying  to charge/3
  no power req if SOC>.999 and trying  to charge/1 -> "Pbty, limited"/1
  Logical Operator1/1 -> [ess_soc_hi_limited], no power req if SOC>.999 and trying  to charge/2
  Relational Operator3/1 -> Logical Operator/2
  Constant9/1 -> Relational Operator3/2, charging (Preq is neg)/2, no power req if SOC<0 and trying  to discharge/3, no power req if SOC>.999 and trying  to charge/1
  Relational Operator/1 -> Logical Operator/1
  Logical Operator2/1 -> [ess_soc_low_limited]

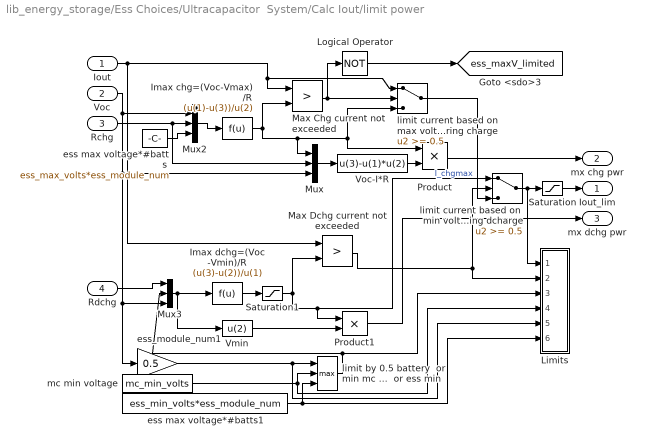
== system lib_energy_storage/Ess Choices/Ultracapacitor  System/Calc Iout/limit power ==
  Iout : Inport
  Voc : Inport  Port=2
  Rchg : Inport  Port=3
  Rdchg : Inport  Port=4
  Imax chg=(Voc-Vmax)/R : Fcn  Expr=(u(1)-u(3))/u(2)
  Imax dchg=(Voc -Vmin)/R : Fcn  Expr=(u(3)-u(2))/u(1)
  Limits : Subsystem
  Logical Operator : Logic  Operator=NOT
  Max Chg current not exceeded : RelationalOperator  Operator=>  InputSameDT=on
  Max Dchg current not exceeded : RelationalOperator  Operator=>  InputSameDT=on
  Mux : Mux  Inputs=3
  Mux2 : Mux  Inputs=3
  Mux3 : Mux  Inputs=3
  Product : Product  SaturateOnIntegerOverflow=on  RndMeth=Zero  InputSameDT=on  OutDataTypeStr=Inherit: Same as first input
  Product1 : Product  SaturateOnIntegerOverflow=on  RndMeth=Zero  InputSameDT=on  OutDataTypeStr=Inherit: Same as first input
  Saturation : Saturate  UpperLimit=625*ess_parallel_mod_num  LowerLimit=-625*ess_parallel_mod_num
  Saturation1 : Saturate  UpperLimit=inf  LowerLimit=0
  Vmin : Fcn  Expr=u(2)
  Voc-I*R : Fcn  Expr=u(3)-u(1)*u(2)
  ess max voltage*#batts : Constant  Value=ess_max_volts*ess_module_num
  ess max voltage*#batts1 : Constant  Value=ess_min_volts*ess_module_num
  ess_module_num1 : Gain  Gain=0.5  SaturateOnIntegerOverflow=on  OutDataTypeStr=Inherit: Same as input  ParamDataTypeStr=Inherit: Same as input
  limit by 0.5 battery  or min mc voltage  or ess min : MinMax  Function=max  Inputs=3  SaturateOnIntegerOverflow=on  InputSameDT=on
  limit current based on  max voltage during charge : Switch  Threshold=0.5  SaturateOnIntegerOverflow=on  InputSameDT=on
  limit current based on  min voltage during dcharge : Switch  Threshold=0.5  SaturateOnIntegerOverflow=on  InputSameDT=on
  mc min voltage : Constant  Value=mc_min_volts
  Iout_lim : Outport
  mx chg pwr : Outport  Port=2
  mx dchg pwr : Outport  Port=3
  tag scope: ess_maxV_limited=global
  wires:
  Mux2/1 -> Imax chg=(Voc-Vmax)/R/1
  Iout/1 -> Max Chg current not exceeded/1, limit current based on  max voltage during charge/1, Max Dchg current not exceeded/1
  Imax chg=(Voc-Vmax)/R/1 -> Max Chg current not exceeded/2, Mux/1, limit current based on  max voltage during charge/3, Product/1
  Rchg/1 -> Mux2/2, Mux/2
  Voc/1 -> Mux2/1, Mux/3, Mux3/3, ess_module_num1/1
  Mux/1 -> Voc-I*R/1
  Voc-I*R/1 -> Product/2
  Product/1 -> mx chg pwr/1
  Max Chg current not exceeded/1 -> limit current based on  max voltage during charge/2, Logical Operator/1
  Logical Operator/1 -> [ess_maxV_limited]
  ess max voltage*#batts/1 -> Mux2/3
  limit current based on  max voltage during charge/1 -> limit current based on  min voltage during dcharge/3  "I_chgmax"
  limit current based on  min voltage during dcharge/1 -> Saturation/1, Limits/1(current req)
  Mux3/1 -> Imax dchg=(Voc -Vmin)/R/1, Vmin/1
  Imax dchg=(Voc -Vmin)/R/1 -> Saturation1/1
  ess max voltage*#batts1/1 -> limit by 0.5 battery  or min mc voltage  or ess min/3, Limits/6(V ess_min_volts)
  Rdchg/1 -> Mux3/1
  Max Dchg current not exceeded/1 -> limit current based on  min voltage during dcharge/2, Limits/2(current bat limited)
  mc min voltage/1 -> limit by 0.5 battery  or min mc voltage  or ess min/2, Limits/4(V mc_min_volts)
  ess_module_num1/1 -> limit by 0.5 battery  or min mc voltage  or ess min/1, Limits/5(V battery (.5Voc))
  limit by 0.5 battery  or min mc voltage  or ess min/1 -> Limits/3(V used), Mux3/2
  Vmin/1 -> Product1/2
  Product1/1 -> mx dchg pwr/1
  Saturation/1 -> Iout_lim/1
  Saturation1/1 -> Max Dchg current not exceeded/2, Product1/1, limit current based on  min voltage during dcharge/1

== system lib_energy_storage/Ess Choices/Ultracapacitor  System/ess tmp/Block NOTES ==
  note: This block models the thermal behavior of a battery module with active air cooling.
      | The module is modeled as a single lumped thermal mass.
      | The fan is on whenever the battery temp is > the set temp.

== system lib_energy_storage/Ess Choices/Ultracapacitor  System/ess tmp/Tair,ave ==
  Qess_case : Inport
  Enable : EnablePort  StatesWhenEnabling=reset
  Block NOTES : Subsystem
      mask Display: disp('Block\nNOTES')
  Tamb-(Q/mcp)/2 : Fcn  Expr=amb_tmp - (u(1)/(ess_mod_airflow*air_cp))/2
  do ex calcs?1 : Constant  Value=ess_th_res_on
  Tair_ave : Outport  OutputWhenDisabled=reset  InitialOutput=amb_tmp
  Th Res : Outport  Port=2  OutputWhenDisabled=reset  InitialOutput=ess_th_res_off
  wires:
  Tamb-(Q/mcp)/2/1 -> Tair_ave/1
  Qess_case/1 -> Tamb-(Q/mcp)/2/1
  do ex calcs?1/1 -> Th Res/1

== system lib_energy_storage/Ess Choices/energy storage <ess>/ess tmp/Block NOTES ==
  note: This block models the thermal behavior of a battery module with active air cooling.
      | The module is modeled as a single lumped thermal mass.
      | The fan is on whenever the battery temp is > the set temp.

== system lib_energy_storage/Ess Choices/energy storage <ess>/ess tmp/Tair,ave ==
  Qess_case : Inport
  Qess_case1 : Inport  Port=2
  Enable : EnablePort  StatesWhenEnabling=reset
  Block NOTES : Subsystem
      mask Display: disp('Block\nNOTES')
  Tamb-(Q/mcp)/1 : Fcn  Expr=amb_tmp - (u(1)/(ess_mod_airflow*air_cp))/2
  Tamb-(Q/mcp)/2 : Fcn  Expr=amb_tmp - (u(1)/(ess_mod_airflow*air_cp))/2
  do ex calcs?1 : Constant  Value=ess_th_res_on
  Tair_ave : Outport  OutputWhenDisabled=reset  InitialOutput=amb_tmp
  Th Res : Outport  Port=2  OutputWhenDisabled=reset  InitialOutput=ess_th_res_off
  Tair : Outport  Port=3  InitialOutput=amb_tmp
  wires:
  do ex calcs?1/1 -> Th Res/1
  Qess_case/1 -> Tamb-(Q/mcp)/2/1
  Tamb-(Q/mcp)/2/1 -> Tair_ave/1
  Qess_case1/1 -> Tamb-(Q/mcp)/1/1
  Tamb-(Q/mcp)/1/1 -> Tair/1

== system lib_energy_storage/Ess Choices/energy storage <ess>/limit power/Limits ==
  SOC  high limited : Inport
  not SOC  low limited : Inport  Port=2
  power req : Inport  Port=3
  power bat limited : Inport  Port=4
  V used : Inport  Port=5
  V mc_min_volts : Inport  Port=6
  V battery (.5Voc) : Inport  Port=7
  V ess_min_volts : Inport  Port=8
  Logical Operator1 : Logic  Operator=NOT  Inputs=1
  Relational Operator{1,3..5} (4 alike) : RelationalOperator  Operator===  InputSameDT=on
  limited by battery : Logic
  limited by battery min V : Logic
  limited by motor controller : Logic
  tag scope: ess_minV_limited=global, ess_pwr_limited=global, ess_soc_hi_limited=global, ess_soc_low_limited=global, mc_voltage_limited=global
  wires:
  SOC  high limited/1 -> [ess_soc_hi_limited]
  not SOC  low limited/1 -> Logical Operator1/1
  Logical Operator1/1 -> [ess_soc_low_limited]
  power req/1 -> Relational Operator1/1
  Relational Operator5/1 -> limited by battery min V/2
  Relational Operator4/1 -> limited by battery/2
  Relational Operator1/1 -> limited by battery min V/1, limited by battery/1, limited by motor controller/1
  Relational Operator3/1 -> limited by motor controller/2
  limited by battery min V/1 -> [ess_minV_limited]
  limited by battery/1 -> [ess_pwr_limited]
  limited by motor controller/1 -> [mc_voltage_limited]
  V ess_min_volts/1 -> Relational Operator5/2
  V battery (.5Voc)/1 -> Relational Operator4/2
  V used/1 -> Relational Operator5/1, Relational Operator4/1, Relational Operator3/1
  V mc_min_volts/1 -> Relational Operator3/2
  power bat limited/1 -> Relational Operator1/2

== system lib_energy_storage/Ess Choices/energy storage <ess>/max pack pwr (W)1/Rchg (ohms)1 ==
  x0 : Inport
  y0 : Inport  Port=2
  Mux : Mux  Inputs=2
  S-function : S-Function  FunctionName=sftable2  Parameters=xindex, yindex, table  EnableBusSupport=off
  table out : Outport  InitialOutput=0
  wires:
  y0/1 -> Mux/2
  S-function/1 -> table out/1
  x0/1 -> Mux/1
  Mux/1 -> S-function/1

== system lib_energy_storage/Ess Choices/energy storage <ess>/max pack pwr (W)1/Rdis (ohms) ==
  x0 : Inport
  y0 : Inport  Port=2
  Mux : Mux  Inputs=2
  S-function : S-Function  FunctionName=sftable2  Parameters=xindex, yindex, table  EnableBusSupport=off
  table out : Outport  InitialOutput=0
  wires:
  y0/1 -> Mux/2
  S-function/1 -> table out/1
  x0/1 -> Mux/1
  Mux/1 -> S-function/1

== system lib_energy_storage/Ess Choices/energy storage <ess>/max pack pwr (W)1/VOC (V) ==
  x0 : Inport
  y0 : Inport  Port=2
  Mux : Mux  Inputs=2
  S-function : S-Function  FunctionName=sftable2  Parameters=xindex, yindex, table  EnableBusSupport=off
  table out : Outport  InitialOutput=0
  wires:
  y0/1 -> Mux/2
  S-function/1 -> table out/1
  x0/1 -> Mux/1
  Mux/1 -> S-function/1

== system lib_energy_storage/Ess Choices/energy storage <ess>/pack Voc, Rint/Rchg (ohms) ==
  x0 : Inport
  y0 : Inport  Port=2
  Mux : Mux  Inputs=2
  S-function : S-Function  FunctionName=sftable2  Parameters=xindex, yindex, table  EnableBusSupport=off
  table out : Outport  InitialOutput=0
  wires:
  Mux/1 -> S-function/1
  x0/1 -> Mux/1
  S-function/1 -> table out/1
  y0/1 -> Mux/2

== system lib_energy_storage/Ess Choices/energy storage <ess>/pack Voc, Rint/Rdis (ohms) ==
  x0 : Inport
  y0 : Inport  Port=2
  Mux : Mux  Inputs=2
  S-function : S-Function  FunctionName=sftable2  Parameters=xindex, yindex, table  EnableBusSupport=off
  table out : Outport  InitialOutput=0
  wires:
  Mux/1 -> S-function/1
  x0/1 -> Mux/1
  S-function/1 -> table out/1
  y0/1 -> Mux/2

== system lib_energy_storage/Ess Choices/energy storage <ess>/pack Voc, Rint/VOC (V) ==
  x0 : Inport
  y0 : Inport  Port=2
  Mux : Mux  Inputs=2
  S-function : S-Function  FunctionName=sftable2  Parameters=xindex, yindex, table  EnableBusSupport=off
  table out : Outport  InitialOutput=0
  wires:
  Mux/1 -> S-function/1
  x0/1 -> Mux/1
  S-function/1 -> table out/1
  y0/1 -> Mux/2

== system lib_energy_storage/Ess Choices/energy storage <ess> RC/Model Parameters/rc ==
  x0 : Inport
  y0 : Inport  Port=2
  Mux : Mux  Inputs=2
  S-function : S-Function  FunctionName=sftable2  Parameters=xindex, yindex, table  EnableBusSupport=off
  table out : Outport  InitialOutput=0
  wires:
  y0/1 -> Mux/2
  S-function/1 -> table out/1
  x0/1 -> Mux/1
  Mux/1 -> S-function/1

== system lib_energy_storage/Ess Choices/energy storage <ess> RC/Model Parameters/re ==
  x0 : Inport
  y0 : Inport  Port=2
  Mux : Mux  Inputs=2
  S-function : S-Function  FunctionName=sftable2  Parameters=xindex, yindex, table  EnableBusSupport=off
  table out : Outport  InitialOutput=0
  wires:
  Mux/1 -> S-function/1
  x0/1 -> Mux/1
  S-function/1 -> table out/1
  y0/1 -> Mux/2

== system lib_energy_storage/Ess Choices/energy storage <ess> RC/Model Parameters/rt ==
  x0 : Inport
  y0 : Inport  Port=2
  Mux : Mux  Inputs=2
  S-function : S-Function  FunctionName=sftable2  Parameters=xindex, yindex, table  EnableBusSupport=off
  table out : Outport  InitialOutput=0
  wires:
  Mux/1 -> S-function/1
  x0/1 -> Mux/1
  S-function/1 -> table out/1
  y0/1 -> Mux/2

== system lib_energy_storage/Ess Choices/energy storage <ess> RC/Thermal Model of Battery/Block NOTES ==
  note: This block models the thermal behavior of a battery module with active air cooling.
      | The module is modeled as a single lumped thermal mass.
      | The fan is on whenever the battery temp is > the set temp.

== system lib_energy_storage/Ess Choices/energy storage <ess> RC/Thermal Model of Battery/Tair,ave ==
  Qess_case : Inport
  Enable : EnablePort  StatesWhenEnabling=reset
  Block NOTES : Subsystem
      mask Display: disp('Block\nNOTES')
  Tamb-(Q/mcp)/2 : Fcn  Expr=amb_tmp - (u(1)/(ess_mod_airflow*air_cp))/2
  do ex calcs?1 : Constant  Value=ess_th_res_on
  Tair_ave : Outport  OutputWhenDisabled=reset  InitialOutput=amb_tmp
  Th Res : Outport  Port=2  OutputWhenDisabled=reset  InitialOutput=ess_th_res_off
  wires:
  do ex calcs?1/1 -> Th Res/1
  Qess_case/1 -> Tamb-(Q/mcp)/2/1
  Tamb-(Q/mcp)/2/1 -> Tair_ave/1

== system lib_energy_storage/Ess Choices/energy storage <ess> nnet/NNet/Neural Network ==
  "p{1}" : Inport  PortDimensions=2
  Layer 1 : Subsystem
  Layer 2 : Subsystem
  "y{1}" : Outport  InitialOutput=[0;0]
  wires:
  Layer 2/1("a{2}") -> "y{1}"/1
  [feedback1] -> Layer 2/1("a{1} ")
  Layer 1/1("a{1}") -> [feedback1]
  "p{1}"/1 -> Layer 1/1("p{1}")

== system lib_energy_storage/Ess Choices/energy storage <ess> Saber/SOC's/Mean ==
  In : Inport
  Average over  10 modules : Gain  Gain=1/10  SaturateOnIntegerOverflow=on  OutDataTypeStr=Inherit: Same as input  ParamDataTypeStr=Inherit: Same as input
  Sum2 : Sum  Inputs=1  SaturateOnIntegerOverflow=on  InputSameDT=on  OutDataTypeStr=Inherit: Same as first input
  Out : Outport
  wires:
  Sum2/1 -> Average over  10 modules/1
  In/1 -> Sum2/1
  Average over  10 modules/1 -> Out/1

== system lib_energy_storage/Ess Choices/energy storage <ess> Saber/SOC's/stop sim ==
  SOC : Inport
  Enable : EnablePort
  Const : Constant  Value=0.1
  Relational Operator : RelationalOperator  Operator=<  InputSameDT=on
  Stop Simulation : Stop
  wires:
  Const/1 -> Relational Operator/2
  SOC/1 -> Relational Operator/1
  Relational Operator/1 -> Stop Simulation/1

== system lib_energy_storage/Ess Choices/energy storage <ess> Saber/Temps/Mean ==
  In : Inport
  Average over  10 modules : Gain  Gain=1/10  SaturateOnIntegerOverflow=on  OutDataTypeStr=Inherit: Same as input  ParamDataTypeStr=Inherit: Same as input
  Sum2 : Sum  Inputs=1  SaturateOnIntegerOverflow=on  InputSameDT=on  OutDataTypeStr=Inherit: Same as first input
  Out : Outport
  wires:
  Sum2/1 -> Average over  10 modules/1
  In/1 -> Sum2/1
  Average over  10 modules/1 -> Out/1

== system lib_energy_storage/Ess Choices/energy storage <ess> Saber/Time Dependent Power Request/Enabled Subsystem1 ==
  In1 : Inport
  Enable : EnablePort
  Out1 : Outport
  wires:
  In1/1 -> Out1/1

== system lib_energy_storage/Ess Choices/energy storage <ess> fundamental model/ess tmp/Block NOTES ==
  note: This block models the thermal behavior of a battery module with active air cooling.
      | The module is modeled as a single lumped thermal mass.
      | The fan is on whenever the battery temp is > the set temp.

== system lib_energy_storage/Ess Choices/energy storage <ess> fundamental model/ess tmp/Tair,ave ==
  Qess_case : Inport
  Enable : EnablePort  StatesWhenEnabling=reset
  Block NOTES : Subsystem
      mask Display: disp('Block\nNOTES')
  Tamb-(Q/mcp)/2 : Fcn  Expr=amb_tmp - (u(1)/(ess_mod_airflow*air_cp))/2
  do ex calcs?1 : Constant  Value=ess_th_res_on
  Tair_ave : Outport  OutputWhenDisabled=reset  InitialOutput=amb_tmp
  Th Res : Outport  Port=2  OutputWhenDisabled=reset  InitialOutput=ess_th_res_off
  wires:
  do ex calcs?1/1 -> Th Res/1
  Qess_case/1 -> Tamb-(Q/mcp)/2/1
  Tamb-(Q/mcp)/2/1 -> Tair_ave/1

== system lib_energy_storage/Ess Choices/energy storage <ess> optima fundamental model/ess tmp/Block NOTES ==
  note: This block models the thermal behavior of a battery module with active air cooling.
      | The module is modeled as a single lumped thermal mass.
      | The fan is on whenever the battery temp is > the set temp.
